simulink model "Second_Simulation"  (R2020a)
settings: Solver=VariableStepAuto  StartTime=0.0  StopTime=1  RelTol=1e-3
libraries: powerlib x6, powerlib_meascontrol x5
settings Model: Creator=amnja  LastModifiedBy=amnja

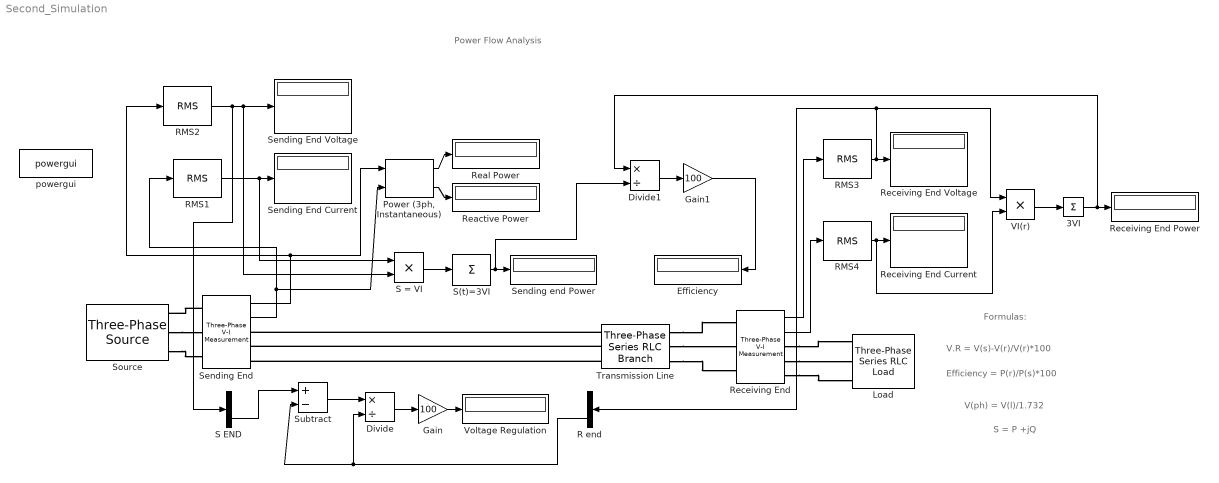
== system Second_Simulation ==
  note: S = P +jQ
  note: V(ph) = V(l)/1.732
  note: Efficiency = P(r)/P(s)*100
  note: V.R = V(s)-V(r)/V(r)*100
  note: Formulas:
  note: Power Flow Analysis
  3VI : Sum  Inputs=+
  Divide : Product  Inputs=*/
  Divide1 : Product  Inputs=*/
  Efficiency : Display
  Gain : Gain  Gain=100
  Gain1 : Gain  Gain=100
  Load : powerlib/Elements/Three-Phase Series RLC Load  LConnTagsString=A|B|C  Configuration=Y (grounded)  NominalVoltage=220e3  Vabc=[1e3 1e3 1e3]  Vabcp=[1e3 1e3 1e3]  NominalFrequency=60  UnbalancedPower=off  ActivePower=304.8e6  InductivePower=228.6e6  CapacitivePower=0  Pabc=[10e3 9e3 11e3]  QLabc=[100 90 110]  QCabc=[100 90 110]  Pabcp=[10e3 9e3 11e3]  QLabcp=[100 90 110]  QCabcp=[100 90 110]  Measurements=None  LoadType=constant Z
  "Power (3ph, Instantaneous)" : powerlib_meascontrol/Measurements/Power (3ph, Instantaneous)
  R end : Demux  Outputs=3
  RMS{1..4} (4 alike) : powerlib_meascontrol/Measurements/RMS  TrueRMS=on  Freq=60  RMSInit=0  Ts=0
  Reactive Power : Display
  Real Power : Display
  Receiving End : powerlib/Measurements/Three-Phase V-I Measurement  VoltageMeasurement=phase-to-ground  SetLabelV=off  LabelV=Vabc  Vpu=off  VpuLL=off  CurrentMeasurement=yes  SetLabelI=off  LabelI=Iabc  Ipu=off  Pbase=100e6  Vbase=500e3  OutputType=Complex  PhasorSimulation=off  PSBequivalent=0
  Receiving End Current : Display
  Receiving End Power : Display
  Receiving End Voltage : Display
  S = VI : Product
  S END : Demux  Outputs=3
  S(t)=3VI : Sum  Inputs=+
  Sending End : powerlib/Measurements/Three-Phase V-I Measurement  VoltageMeasurement=phase-to-ground  SetLabelV=off  LabelV=Vabc  Vpu=off  VpuLL=off  CurrentMeasurement=yes  SetLabelI=off  LabelI=Iabc  Ipu=off  Pbase=100e6  Vbase=500e3  OutputType=Complex  PhasorSimulation=off  PSBequivalent=0
  Sending End Current : Display
  Sending End Voltage : Display
  Sending end Power : Display
  Source : powerlib/Electrical Sources/Three-Phase Source  InternalConnection=Yg  VoltagePhases=off  Voltage=250000  PhaseAngle=0  Voltage_phases=[25e3 25e3 25e3]/sqrt(3)  PhaseAngles_phases=[0 -120 +120]  Frequency=60  NonIdealSource=off  SpecifyImpedance=off  Resistance=0.8929  Inductance=16.58e-3  ShortCircuitLevel=100e6  BaseVoltage=25e3  XRratio=7  BusType=swing  Pref=10e3  Qref=0  Prefabc=[10e3, 10e3, 10e3]  Qrefabc=[0, 0, 0]  Qmin=-inf  Qmax=inf
  Subtract : Sum  Inputs=+-
  Transmission Line : powerlib/Elements/Three-Phase Series RLC Branch  LConnTagsString=A|B|C  RConnTagsString=A|B|C  BranchType=RL  Resistance=6  Inductance=0.053052  Capacitance=1e-6  Measurements=None
  VI(r) : Product
  Voltage Regulation : Display
  powergui : powerlib/powergui  Priority=1  SimulationMode=Continuous  SampleTime=50e-6  frequency=60  Iterations=50  frequencyindice=60  Pbase=100e6  ErrMax=1e-4  UnitsV=kV  UnitsW=MW  buscounter=0  FunctionMessages=off  echomessages=off  EnableUseOfTLC=off  CurrentSourceSwitches=off  DisableSnubberDevices=off  DisableRonSwitches=off  DisableVfSwitches=off  DisplayEquations=off  AutomaticDiscreteSolvers=off  SolverType=Tustin/Backward Euler (TBE)  Interpol=off  ExternalGateDelay=off  methode=off  Ts=100  x0status=blocks  SPID=on  SwTol=0  HookPort=off  NonlinearTolerance=1e-4  nMaxIteration=100  ContinueOnMaxIteration=off  RestoreLinks=warning  ResistiveCurrentMeasurement=off  Frange=[0:2:500]  Ylog=off  Xlog=on  ShowGrid=off  save=off  variable=ZData  structure=0  ZoomFFT=off  StartTime=0.0  cycles=1  DisplayStyle=1  fundamental=60  FreqAxis=off  MaxFrequency=1000  frequencyindicesteady=1  RmsSteady=1  display=off
  wires:
  Sending End/1 -> "Power (3ph, Instantaneous)"/1, RMS2/1
  RMS2/1 -> S END/1, Sending End Voltage/1, S = VI/2
  RMS1/1 -> S = VI/1, Sending End Current/1
  Sending End/2 -> "Power (3ph, Instantaneous)"/2, RMS1/1
  "Power (3ph, Instantaneous)"/1 -> Real Power/1
  "Power (3ph, Instantaneous)"/2 -> Reactive Power/1
  S = VI/1 -> S(t)=3VI/1
  S(t)=3VI/1 -> Divide1/2, Sending end Power/1
  Receiving End/1 -> RMS3/1
  RMS3/1 -> R end/1, VI(r)/1, Receiving End Voltage/1
  Receiving End/2 -> RMS4/1
  RMS4/1 -> VI(r)/2, Receiving End Current/1
  VI(r)/1 -> 3VI/1
  3VI/1 -> Divide1/1, Receiving End Power/1
  S END/3 -> Subtract/1
  R end/3 -> Divide/2, Subtract/2
  Subtract/1 -> Divide/1
  Divide/1 -> Gain/1
  Gain/1 -> Voltage Regulation/1
  Divide1/1 -> Gain1/1
  Gain1/1 -> Efficiency/1
  connections:
  Sending End/LConn1 -- Source/RConn1
  Source/RConn2 -- Sending End/LConn2
  Source/RConn3 -- Sending End/LConn3
  Transmission Line/LConn1 -- Sending End/RConn1
  Transmission Line/LConn2 -- Sending End/RConn2
  Transmission Line/LConn3 -- Sending End/RConn3
  Transmission Line/RConn1 -- Receiving End/LConn1
  Transmission Line/RConn2 -- Receiving End/LConn2
  Transmission Line/RConn3 -- Receiving End/LConn3
  Receiving End/RConn1 -- Load/LConn1
  Receiving End/RConn2 -- Load/LConn2
  Receiving End/RConn3 -- Load/LConn3
